simulink model "BMS_BIL_Wrapper"  (R2025b)
settings: Solver=FixedStepAuto  StartTime=0.0  StopTime=10.0  RelTol=1e-3  EnableMultiTasking=on
InitFcn:
  | battery_init;
  | Full_Charge_Volt=4.2; % unit volts
  | Cutoff_Volt=3; % unit volts
  | Delta=.02;
  | ContactorTime=20;
  | ContactorTimeOut=100;
  | High_TempLim=333;
  | Low_TempLim=253;
  | Sensor_Fault_Treshold=.02;
  | CurrentTimeout=1;
  | Allowed_Delta=.04;
  | Bal_On_Time=30;
  | Bal_Off_Time=5;
  | BalNotAct_Time=10;
values from neighbouring files (symbols this model uses):
  ADC_Volt_Resolution = .000089    (= 8.9e-05)    [MCU.m]
  bonka_R0 = [ ... (first row only)    [battery_init.m]
  bonka_SOC = [0, 0.1, 0.2, 0.3, 0.4, 0.5, 0.6, 0.7, 0.8, 0.9, 1.0]    [battery_init.m]
  bonka_T = [263.15, 273.15, 298.15, 313.15, 328.15]    [battery_init.m]
  Capacity = 5.200    (= 5.2)    [MCU.m]
  Charge_Rate = 1    [battery_init.m]
  Discharge_Rate = -1    [battery_init.m]
  R_NTC = 10000    [MCU.m]
  R_Pullup = 10000    [MCU.m]
  R_Sense = .01    (= 0.01)    [MCU.m]
  V_Bat_Div_Res = .00133    (= 0.00133)    [MCU.m]
  V_ISENSE_Res = .00000133    (= 1.33e-06)    [MCU.m]
undefined symbols (not defined in the file or in its folder): DiscIntNeverNeededParam
libraries: simulink x58, stm32f4xxblockslib x1, stm32blockslib x1
(part 2 of 2)

== matlab function BMS_BIL_Wrapper/Data_Acquisition_From_L99BM114/All_Frames/Subsystem/Subsystem/MATLAB Function ==
  data: u input size=[1 34]; crc output size=[1 6]
function crc = calc_crc6_34(u)
%#codegen
% Inputs:
%   u   - A 34-element logical or binary array representing the message bits (MSB first).
% Outputs:
%   crc - A 6-element logical array containing the computed 6-bit CRC.

% 1. Define configuration parameters
% Seed: '111000'
seed = logical([1, 1, 1, 0, 0, 0]); 

% Polynomial: x^6 + x^4 + x^3 + 1 -> Binary 1011001. 
% For shift register logic, drop the highest coefficient (x^6):
poly = logical([0, 1, 1, 0, 0, 1]); 

% 2. Initialize internal shift register with seed
reg = seed;

% 3. Process each bit of the 34-bit input frame (Standard Direct Algorithm)
for i = 1:34
    % Determine if a reduction/XOR is needed based on the outgoing bit
    xor_bit = xor(reg(1), u(i));
    
    % Shift left by 1 position
    reg = [reg(2:6), false];
    
    % Apply polynomial if the XOR condition is true
    if xor_bit
        reg = xor(reg, poly);
    end
end
crc=reg;

== stateflow chart BMS_BIL_Wrapper/BMS_Control/Subsystem1/Chart ==
  state Balancing_Off
    en:
    Bal_Cmd(:,:)= false;
    en, du:
    DeltaCellVolt=Max_Voltage-Min_Voltage;
  state Balancing_On
    en, du:
    DeltaCellVolt=Max_Voltage-Min_Voltage;
    state Balance_Active
      en, du:
      Bal_Cmd=((Vmod-Min_Voltage)> Allowed_Delta/2)';
      flgBalCompl=all(~Bal_Cmd);
    state Balance_Not_Active
    (default) -> Balance_Active
    Balance_Not_Active -> Balance_Active [order 1] : [after(BalNotAct_Time, sec) &&...
        |  DeltaCellVolt> Allowed_Delta]
    Balance_Active -> Balance_Not_Active : [flgBalCompl]
  (default) -> Balancing_Off : {flgBalCompl=true}
  Balancing_Off -> Balancing_On : [flgBalInt &&...
      | BMS_State_Out==BMS_State.Charging &&...
      | after(Bal_Off_Time, sec) &&...
      | DeltaCellVolt> Allowed_Delta]
  Balancing_On -> Balancing_Off : [BMS_State_Out==BMS_State.Flying]
  Balance_Not_Active -> Balancing_Off [order 2] : [after(Bal_On_Time, sec)]
  data: BMS_State_Out input; Min_Voltage input single; Max_Voltage input single; Bal_Cmd output boolean; Allowed_Delta parameter single; DeltaCellVolt local single; Bal_On_Time parameter single; Bal_Off_Time parameter single; BalNotAct_Time parameter single; Vmod input single; flgBalCompl local boolean =false; flgBalInt local =true

== matlab function BMS_BIL_Wrapper/Data_Acquisition_From_L99BM114/All_Frames/Subsystem/Subsystem/MATLAB Function1 ==
  data: u_1 input size=[1 34]; crc_1 output size=[1 6]
function crc_1 = calc_crc6_34_1(u_1)
%#codegen
% Inputs:
%   u   - A 34-element logical or binary array representing the message bits (MSB first).
% Outputs:
%   crc - A 6-element logical array containing the computed 6-bit CRC.

% 1. Define configuration parameters
% Seed: '111000'
seed = logical([1, 1, 1, 0, 0, 0]); 

% Polynomial: x^6 + x^4 + x^3 + 1 -> Binary 1011001. 
% For shift register logic, drop the highest coefficient (x^6):
poly = logical([0, 1, 1, 0, 0, 1]); 

% 2. Initialize internal shift register with seed
reg = seed;

% 3. Process each bit of the 34-bit input frame (Standard Direct Algorithm)
for i = 1:34
    % Determine if a reduction/XOR is needed based on the outgoing bit
    xor_bit = xor(reg(1), u_1(i));
    
    % Shift left by 1 position
    reg = [reg(2:6), false];
    
    % Apply polynomial if the XOR condition is true
    if xor_bit
        reg = xor(reg, poly);
    end
end
crc_1 = reg;
